simulink model "EPS_sim_test_v3"  (R2020b)
settings: Solver=FixedStepAuto  StartTime=0.0  StopTime=tsimulation  FixedStep=delta_t  MaxStep=10  RelTol=1e-3
values from neighbouring files (symbols this model uses):
  C = Cbat*Nbp*3600    (= 37440)    [demoEPS.m]    (also in demoEPS_R2019a.m; demoEPS_v1.m; demoEPS_v1a.m; demoEPS_v1test.m)
  DOD_0 = 0    [demoEPS.m]    (also in demoEPS_R2019a.m; demoEPS_v1.m; demoEPS_v1a.m; demoEPS_v1test.m)
  eff_iBat = 0.95    [demoEPS_v3.m]    (also in demoEPS_v4.m; demoEPS_v5.m)
  I_BC_max = -input (4)    [battchargedischarge.m]    (also in demoEPS.m = 3; demoEPS_R2019a.m = 3; demoEPS_v1.m = 3; demoEPS_v1a.m = 3)
  I_BD_max = input (3)    [battchargedischarge.m]    (also in demoEPS.m = 5; demoEPS_R2019a.m = 5; demoEPS_v1.m = 5; demoEPS_v1a.m = 5)
  Nbs = math.ceil(Vbusmin/Vbatmin)    [calc_mass_EPS.m]    (also in demoEPS.m = 4; demoEPS_R2019a.m = 4; demoEPS_v1.m = 4; demoEPS_v1a.m = 4)
  P_eps = 0.6    [demoEPS.m]    (also in demoEPS_R2019a.m; demoEPS_v1.m; demoEPS_v1a.m; demoEPS_v1test.m)
  Pload1 = 50    [demoEPS.m]    (also in demoEPS_R2019a.m; demoEPS_v1.m; demoEPS_v1a.m; demoEPS_v1test.m)
  Pload2 = 2    [demoEPS.m]    (also in demoEPS_R2019a.m; demoEPS_v1.m; demoEPS_v1a.m; demoEPS_v1test.m)
  Pload3 = 2.5    [demoEPS.m]    (also in demoEPS_R2019a.m; demoEPS_v1.m; demoEPS_v1a.m; demoEPS_v1test.m)
  Pload4 = 1.7    [demoEPS.m]    (also in demoEPS_R2019a.m; demoEPS_v1.m; demoEPS_v1a.m; demoEPS_v1test.m)
  Psa = 48    [demoEPS.m]    (also in demoEPS_R2019a.m; demoEPS_v1.m; demoEPS_v1a.m; demoEPS_v1test.m)
  Torbit = 2*pi*sqrt(((h+6378)^3)/398600)/60    [calc_mass_EPS.m]    (also in demoEPS.m = 5400; demoEPS_R2019a.m = 2*pi*sqrt(a^3/(3.986004418E5)); demoEPS_v1.m = 5400; demoEPS_v1a.m = 2*pi*sqrt(a^3/(3.986004418E5)))
libraries: simulink x2
settings Model: Creator=Ricardo  LastModifiedBy=colpari

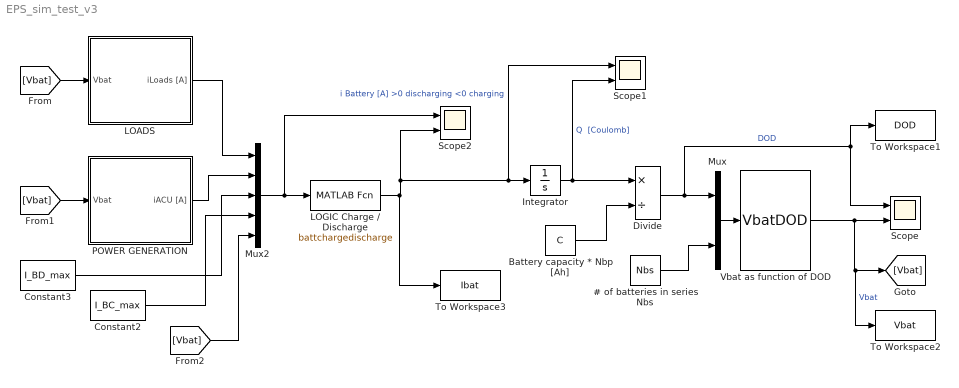
== system EPS_sim_test_v3 ==
  # of batteries in series Nbs : Constant  Value=Nbs
  Battery capacity * Nbp [Ah] : Constant  Value=C
  Constant2 : Constant  Value=I_BC_max
  Constant3 : Constant  Value=I_BD_max
  Divide : Product  Inputs=*/
  Integrator : Integrator  InitialCondition=DOD_0
  LOADS : Subsystem
  LOGIC Charge / Discharge : MATLABFcn  MATLABFcn=battchargedischarge
  Mux : Mux  Inputs=2
  Mux2 : Mux  Inputs=5
  POWER GENERATION : Subsystem
  Scope : Scope  NumInputPorts=2
  Scope1 : Scope  NumInputPorts=2
  Scope2 : Scope  NumInputPorts=2
  To Workspace1 : ToWorkspace  VariableName=DOD  SaveFormat=Timeseries  SampleTime=-1
  To Workspace2 : ToWorkspace  VariableName=Vbat  SaveFormat=Timeseries  SampleTime=-1
  To Workspace3 : ToWorkspace  VariableName=Ibat  SaveFormat=Timeseries  SampleTime=-1
  Vbat as function of DOD : MATLABFcn  MATLABFcn=VbatDOD
  wires:
  Mux/1 -> Vbat as function of DOD/1
  # of batteries in series Nbs/1 -> Mux/2
  Vbat as function of DOD/1 -> To Workspace2/1, [Vbat], Scope/2  "Vbat"
  Divide/1 -> To Workspace1/1, Scope/1, Mux/1  "DOD"
  Integrator/1 -> Scope1/2, Divide/1  "Q  [Coulomb]"
  Battery capacity * Nbp [Ah]/1 -> Divide/2
  [Vbat] -> LOADS/1(Vbat)
  POWER GENERATION/1(iACU [A]) -> Mux2/2
  [Vbat] -> POWER GENERATION/1(Vbat)
  LOADS/1(iLoads [A]) -> Mux2/1
  Mux2/1 -> LOGIC Charge / Discharge/1, Scope2/1
  Constant3/1 -> Mux2/3
  Constant2/1 -> Mux2/4
  LOGIC Charge / Discharge/1 -> To Workspace3/1, Scope1/1, Integrator/1, Scope2/2  "i Battery [A] >0 discharging <0 charging"
  [Vbat] -> Mux2/5

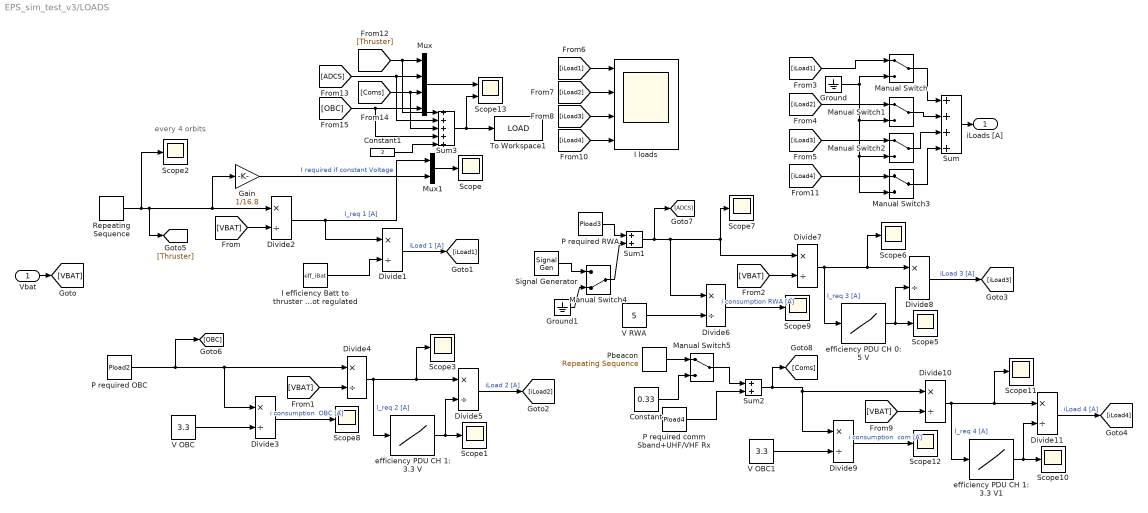
== system EPS_sim_test_v3/LOADS ==
  note: every 4 orbits
  Vbat : Inport
  Constant : Constant  Value=0.33
  Constant1 : Constant  Value=2
  Divide{1..11} (11 alike) : Product  Inputs=*/
  Gain : Gain  Gain=1/16.8
  Ground : Ground
  Ground1 : Ground
  I efficiency Batt to thruster not regulated : Constant  Value=eff_iBat
  I loads : Scope  NumInputPorts=4
  Manual Switch{,1..3,5} (5 alike) : ManualSwitch
  Manual Switch4 : ManualSwitch  CurrentSetting=0
  Mux : Mux
  Mux1 : Mux  Inputs=2
  P required OBC : Constant  Value=Pload2
  P required RWA : Constant  Value=Pload3
  P required comm Sband+UHF/VHF Rx : Constant  Value=Pload4
  Pbeacon : simulink/Sources/Repeating Sequence  rep_seq_t=[0, 1, 21, 22, 200]  rep_seq_y=[0 3.3 3.3 0 0]
  Repeating Sequence : simulink/Sources/Repeating Sequence  rep_seq_t=[0, Torbit-501,Torbit-500, Torbit-300, Torbit-299,Torbit-250,Torbit-249,Torbit-50,Torbit-49, Torbit+1, (Torbit*1.5),(Torbit*1.5)+1, 2*Torbit,3*Torbit]  rep_seq_y="[0.32 0.32 60 60 0.32 0.32  40 40 0.32 Pload1 Pload1 0.32 0.32 0.32]"
  Scope{,1..3,5..12} (12 alike) : Scope
  Scope13 : Scope  NumInputPorts=2
  Signal Generator : SignalGenerator  WaveForm=random  Amplitude=0.6  Frequency=0.01
  Sum : Sum  Inputs=++++
  Sum1 : Sum
  Sum2 : Sum
  Sum3 : Sum  Inputs=+++++
  To Workspace1 : ToWorkspace  VariableName=LOAD  SaveFormat=Timeseries  SampleTime=-1
  V OBC : Constant  Value=3.3
  V OBC1 : Constant  Value=3.3
  V RWA : Constant  Value=5
  efficiency PDU CH 0: 5 V : Lookup_n-D  NumberOfTableDimensions=1  BreakpointsForDimension1=[0,0.15,0.18,0.25,0.4,0.5,0.75,1,1.5,2,3,4]  Table=[0.8,0.8,0.8,0.8,0.85,0.95,0.96,0.958,0.95,0.94,0.92,0.9]  InternalRulePriority=Speed  RndMeth=Simplest  InputSameDT=on
  efficiency PDU CH 1: 3.3 V : Lookup_n-D  NumberOfTableDimensions=1  BreakpointsForDimension1=[0,0.15,0.18,0.25,0.4,0.5,0.75,1,1.5,2,3,4]  Table=[0.94,0.95,0.95,0.95,0.945,0.946,0.945,0.9425,0.931,0.9181,0.8916,0.862]  InternalRulePriority=Speed  RndMeth=Simplest  InputSameDT=on
  efficiency PDU CH 1: 3.3 V1 : Lookup_n-D  NumberOfTableDimensions=1  BreakpointsForDimension1=[0,0.15,0.18,0.25,0.4,0.5,0.75,1,1.5,2,3,4]  Table=[0.94,0.95,0.95,0.95,0.945,0.946,0.945,0.9425,0.931,0.9181,0.8916,0.862]  InternalRulePriority=Speed  RndMeth=Simplest  InputSameDT=on
  iLoads [A] : Outport
  wires:
  Gain/1 -> Mux1/2  "I required if constant Voltage"
  Divide2/1 -> Mux1/1, Divide1/1  "I_req 1 [A]"
  P required OBC/1 -> [OBC], Divide4/1, Divide3/1
  V OBC/1 -> Divide3/2
  Vbat/1 -> [VBAT]
  [VBAT] -> Divide2/2
  [VBAT] -> Divide4/2
  Divide4/1 -> efficiency PDU CH 1: 3.3 V/1, Scope3/1, Divide5/1  "I_req 2 [A]"
  Sum/1 -> iLoads [A]/1
  Mux1/1 -> Scope/1
  efficiency PDU CH 1: 3.3 V/1 -> Scope1/1, Divide5/2
  Repeating Sequence/1 -> Scope2/1, [Thruster], Gain/1, Divide2/1
  I efficiency Batt to thruster not regulated/1 -> Divide1/2
  Divide1/1 -> [iLoad1]  "iLoad 1 [A]"
  Divide5/1 -> [iLoad2]  "iLoad 2 [A]"
  V RWA/1 -> Divide6/2
  Divide7/1 -> efficiency PDU CH 0: 5 V/1, Scope6/1, Divide8/1  "I_req 3 [A]"
  efficiency PDU CH 0: 5 V/1 -> Scope5/1, Divide8/2
  [VBAT] -> Divide7/2
  Divide8/1 -> [iLoad3]  "iLoad 3 [A]"
  Manual Switch/1 -> Sum/1
  Manual Switch1/1 -> Sum/2
  Manual Switch2/1 -> Sum/3
  [iLoad2] -> I loads/2
  [iLoad1] -> I loads/1
  [iLoad3] -> I loads/3
  Sum1/1 -> [ADCS], Divide6/1, Divide7/1, Scope7/1
  P required RWA/1 -> Sum1/1
  Signal Generator/1 -> Manual Switch4/1
  Divide3/1 -> Scope8/1  "i consumption  OBC [A]"
  Divide6/1 -> Scope9/1  "i consumption RWA [A]"
  Divide9/1 -> Scope12/1  "i consumption  com [A]"
  [VBAT] -> Divide10/2
  Divide11/1 -> [iLoad4]  "iLoad 4 [A]"
  efficiency PDU CH 1: 3.3 V1/1 -> Scope10/1, Divide11/2
  Divide10/1 -> efficiency PDU CH 1: 3.3 V1/1, Scope11/1, Divide11/1  "I_req 4 [A]"
  Sum2/1 -> [Coms], Divide9/1, Divide10/1
  V OBC1/1 -> Divide9/2
  [iLoad4] -> I loads/4
  Manual Switch3/1 -> Sum/4
  P required comm Sband+UHF/VHF Rx/1 -> Sum2/2
  Pbeacon/1 -> Manual Switch5/1
  [iLoad4] -> Manual Switch3/1
  [iLoad3] -> Manual Switch2/1
  [iLoad2] -> Manual Switch1/1
  [iLoad1] -> Manual Switch/1
  Ground/1 -> Manual Switch/2, Manual Switch3/2, Manual Switch2/2, Manual Switch1/2
  Manual Switch4/1 -> Sum1/2
  Ground1/1 -> Manual Switch4/2
  Manual Switch5/1 -> Sum2/1
  Constant/1 -> Manual Switch5/2
  Mux/1 -> Scope13/1
  [Thruster] -> Sum3/1, Mux/1
  [ADCS] -> Sum3/2, Mux/2
  [Coms] -> Sum3/3, Mux/3
  [OBC] -> Sum3/4, Mux/4
  Constant1/1 -> Sum3/5
  Sum3/1 -> To Workspace1/1, Scope13/2

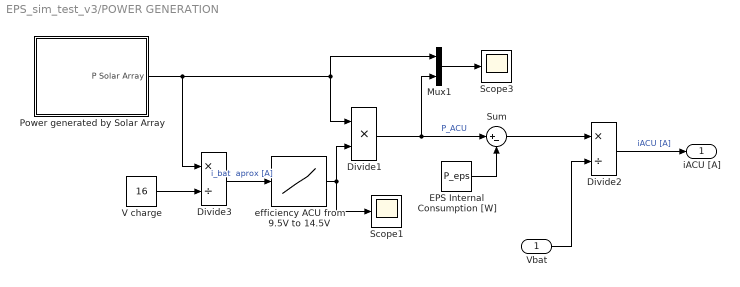
== system EPS_sim_test_v3/POWER GENERATION ==
  Vbat : Inport
  Divide1 : Product  Inputs=**
  Divide2 : Product  Inputs=*/
  Divide3 : Product  Inputs=*/
  EPS Internal Consumption [W] : Constant  Value=P_eps
  Mux1 : Mux  Inputs=2
  Power generated by Solar Array : Subsystem
  Scope1 : Scope
  Scope3 : Scope
  Sum : Sum  Inputs=|+-
  V charge : Constant  Value=16
  efficiency ACU from 9.5V to 14.5V : Lookup_n-D  NumberOfTableDimensions=1  BreakpointsForDimension1=[0,0.13,0.16,0.236,0.4187,0.654,0.684,0.745,0.801,0.9372,1.046,1.16,1.21,1.5,1.66,2,4]  Table=[0.905,0.928,0.9296,0.9296,0.9337,0.9296,0.9296,0.9296,0.9275,0.9275,0.9254,0.9254,0.9234,0.9193,0.9193,0.9134,0.9134]  InternalRulePriority=Speed  RndMeth=Simplest  InputSameDT=on
  iACU [A] : Outport
  wires:
  Divide2/1 -> iACU [A]/1  "iACU [A]"
  Mux1/1 -> Scope3/1
  Vbat/1 -> Divide2/2
  efficiency ACU from 9.5V to 14.5V/1 -> Scope1/1, Divide1/2
  Divide1/1 -> Sum/1, Mux1/2  "P_ACU"
  Sum/1 -> Divide2/1
  EPS Internal Consumption [W]/1 -> Sum/2
  Divide3/1 -> efficiency ACU from 9.5V to 14.5V/1  "i_bat  aprox [A]"
  V charge/1 -> Divide3/2
  Power generated by Solar Array/1(P Solar Array) -> Divide3/1, Divide1/1, Mux1/1

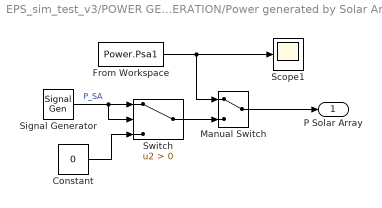
== system EPS_sim_test_v3/POWER GENERATION/Power generated by Solar Array ==
  Constant : Constant  Value=0
  From Workspace : FromWorkspace  VariableName=Power.Psa1
  Manual Switch : ManualSwitch
  Scope1 : Scope
  Signal Generator : SignalGenerator  Amplitude=-Psa  Frequency=1/Torbit
  Switch : Switch  Criteria=u2 > Threshold
  P Solar Array : Outport
  wires:
  From Workspace/1 -> Manual Switch/1, Scope1/1
  Constant/1 -> Switch/3
  Signal Generator/1 -> Switch/2, Switch/1  "P_SA"
  Manual Switch/1 -> P Solar Array/1
  Switch/1 -> Manual Switch/2
